simulink model "kalman_vision_slow"  (R2013a)
settings: Solver=ode3  StartTime=0.0  StopTime=Inf  FixedStep=ts  RelTol=1e-3
InitFcn:
  | ts=1/30
undefined symbols (not defined in the file or in its folder): gray, none, serial, videoinput
libraries: simulink x6, visionsinks x2, visionstatistics x1, imaqlib x1, visiontextngfix x1, instrumentlib x1
settings Model: Creator=Michael  LastModifiedBy=nano

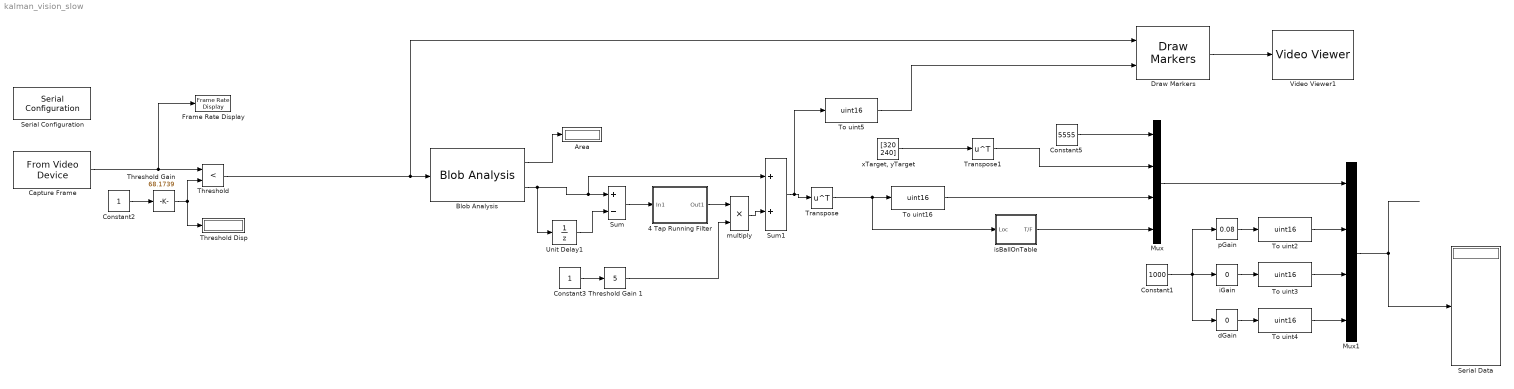
== system kalman_vision_slow ==
  "4 Tap Running Filter " : Subsystem
  Area : Display
  Blob Analysis : visionstatistics/Blob Analysis  Tag=vipblks_row_conv  area=on  centroid=on  bBox=off  majorAxis=off  minorAxis=off  angle=off  eccentricity=off  equivDiameterSq=off  extent=off  perimeter=off  maxBlobs=1  warnIfNumBlobsExceeded=off  isCount=off  useMinArea=off  minArea=500  useMaxArea=on  maxArea=5000  excludeBorderBlob=on  outDT=double  isOutVarDim=off  isFill=on  fillValues=-1  conn=8  isLabel=off  outputMode=Binary point scaling  outputWordLength=32  outputFracLength=16  firstCoeffMode=Binary point scaling  firstCoeffWordLength=16  firstCoeffFracLength=14  secondCoeffMode=Binary point scaling  secondCoeffWordLength=32  secondCoeffFracLength=16  accumMode=Binary point scaling  accumWordLength=32  accumFracLength=0  prodOutputMode=Binary point scaling  prodOutputWordLength=32  prodOutputFracLength=16  roundingMode=Floor  overflowMode=off
  Capture Frame : imaqlib/From Video Device  DeviceMenu=winvideo 1 (HP Prem AF Webcam KQ245AA)  Device=winvideo 1 (HP Prem AF Webcam KQ245AA)  ObjConstructor=videoinput('winvideo', 1)  VideoFormatMenu=MJPG_640x480  VideoFormat=MJPG_640x480  VideoSource=input1  ROIPosition=[0 0 480 640]  EnableHWTrigger=off  TriggerConfiguration=none/none  SampleTime=1/30  OutputPortsMode=One multidimensional signal  DataType=uint8  CanDoHWTrigger=no  ReturnedColorSpace=grayscale  BlockHandle=1913.0001  ROIWidth=640  ROIHeight=480  ROIColumn=0  ROIRow=0  EngXMLPath=C:\Program Files\MATLAB\R2013a\toolbox\imaq\imaq\private  DevXMLPath=C:\Program Files\MATLAB\R2013a\toolbox\imaq\imaqadaptors\win64  EngLibPath=C:\Program Files\MATLAB\R2013a\toolbox\imaq\imaqblks\imaqmex\win64  ColorSpace=grayscale  BayerSensorAlignment=grbg
  Constant1 : Constant  Value=1000  OutDataTypeStr=double
  Constant2 : Constant  OutDataTypeStr=double
  Constant3 : Constant  OutDataTypeStr=double
  Constant5 : Constant  Value=5555  OutDataTypeStr=uint16
  Draw Markers : visiontextngfix/Draw Markers  shape=Plus  size=40  fill=off  fillClrSource=Specify via dialog  display=White  intensity=200  color=[150 0 0]  opacity=0.6  viewport=Entire image  antialiasing=off  inType=Obsolete  imagePorts=One multidimensional signal  prodOutputMode=Binary point scaling  prodOutputWordLength=32  prodOutputFracLength=14  memoryMode=Specify word length  memoryWordLength=16  memoryFracLength=15  roundingMode=Floor  overflowMode=off
  Frame Rate Display : visionsinks/Frame Rate Display  UpdateRate=30
  Mux : Mux
  Mux1 : Mux
  Serial Configuration : instrumentlib/Serial Configuration  Priority=-200000  ComPortMenu=COM7  ComPort=COM7  ObjConstructor=serial('COM7');  BaudRate=115200  DataBits=8  Parity=none  StopBits=1  FlowControl=none  Timeout=10  ByteOrder=LittleEndian
  Serial Data : Display
  Sum : Sum  Inputs=+-
  Sum1 : Sum
  Threshold : RelationalOperator  Operator=<  OutDataTypeStr=boolean  ZeroCross=off
  "Threshold Gain " : simulink/Math Operations/Slider Gain  low=0  gain=68.1739  high=258
  Threshold Gain 1 : simulink/Math Operations/Slider Gain  low=0  gain=5  high=30
  Threshold Disp : Display
  To uint{2..5,16} (5 alike) : DataTypeConversion  OutDataTypeStr=uint16
  Transpose : Math  Operator=transpose  SaturateOnIntegerOverflow=on
  Transpose1 : Math  Operator=transpose  SaturateOnIntegerOverflow=on
  Unit Delay1 : UnitDelay  SampleTime=-1
  Video Viewer1 : visionsinks/Video Viewer  inputType=Obsolete7b  imagePorts=One multidimensional signal  useColorMap=off  colormapValue=gray(256)  specRange=off  minInputVal=0  maxInputVal=255  FigPos=[151 864 821 605]  AxisZoom=on  trueSizedOnce=off  OpenAtMdlStart=on  DefaultConfigurationName=vipscopes.VideoViewerScopeCfg
  dGain : simulink/Math Operations/Slider Gain  low=0  gain=0  high=1.5
  iGain : simulink/Math Operations/Slider Gain  low=0  gain=0  high=1
  isBallOnTable : Subsystem
  "multiply " : Product  Inputs=**
  pGain : simulink/Math Operations/Slider Gain  low=0  gain=0.08  high=5
  "xTarget, yTarget" : Constant  Value=[320 240]  VectorParams1D=off  OutDataTypeStr=uint16
  wires:
  Blob Analysis/1 -> Area/1
  Threshold/1 -> Draw Markers/1, Blob Analysis/1
  Transpose/1 -> isBallOnTable/1(Loc), To uint16/1
  Draw Markers/1 -> Video Viewer1/1
  Capture Frame/1 -> Frame Rate Display/1, Threshold/1
  isBallOnTable/1(T/F) -> Mux/4
  To uint16/1 -> Mux/3
  Transpose1/1 -> Mux/2
  Constant5/1 -> Mux/1
  pGain/1 -> To uint2/1
  iGain/1 -> To uint3/1
  dGain/1 -> To uint4/1
  Constant1/1 -> dGain/1, iGain/1, pGain/1
  To uint2/1 -> Mux1/2
  To uint3/1 -> Mux1/3
  To uint4/1 -> Mux1/4
  Constant2/1 -> "Threshold Gain "/1
  "Threshold Gain "/1 -> Threshold/2, Threshold Disp/1
  Mux/1 -> Mux1/1
  Mux1/1 -> Serial Data/1
  Unit Delay1/1 -> Sum/2
  Constant3/1 -> Threshold Gain 1/1
  Threshold Gain 1/1 -> "multiply "/2
  Sum/1 -> "4 Tap Running Filter "/1(In1)
  "multiply "/1 -> Sum1/2
  "xTarget, yTarget"/1 -> Transpose1/1
  "4 Tap Running Filter "/1(Out1) -> "multiply "/1
  Sum1/1 -> To uint5/1, Transpose/1
  Blob Analysis/2 -> Unit Delay1/1, Sum1/1, Sum/1
  To uint5/1 -> Draw Markers/2

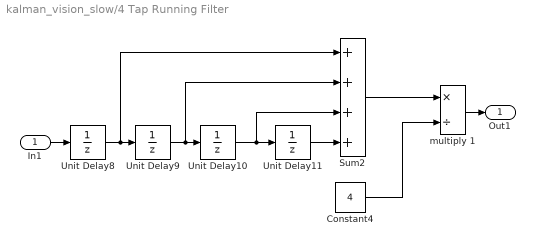
== system kalman_vision_slow/4 Tap Running Filter  ==
  In1 : Inport
  Constant4 : Constant  Value=4  OutDataTypeStr=double
  Sum2 : Sum  Inputs=++++
  Unit Delay{8..11} (4 alike) : UnitDelay  SampleTime=-1
  multiply 1 : Product  Inputs=*/
  Out1 : Outport
  wires:
  Unit Delay8/1 -> Sum2/1, Unit Delay9/1
  Constant4/1 -> multiply 1/2
  Unit Delay11/1 -> Sum2/4
  In1/1 -> Unit Delay8/1
  multiply 1/1 -> Out1/1
  Unit Delay10/1 -> Sum2/3, Unit Delay11/1
  Sum2/1 -> multiply 1/1
  Unit Delay9/1 -> Sum2/2, Unit Delay10/1

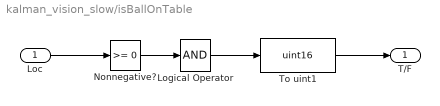
== system kalman_vision_slow/isBallOnTable ==
  Loc : Inport
  Logical Operator : Logic  Inputs=1  AllPortsSameDT=off  OutDataTypeStr=boolean
  Nonnegative? : simulink/Logic and Bit Operations/Compare To Zero  relop=>=  OutDataTypeStr=boolean  ZeroCross=off
  To uint1 : DataTypeConversion  OutDataTypeStr=uint16
  T/F : Outport
  wires:
  Logical Operator/1 -> To uint1/1
  Nonnegative?/1 -> Logical Operator/1
  To uint1/1 -> T/F/1
  Loc/1 -> Nonnegative?/1
